simulink library "Math"  (R2023a)
settings: Solver=VariableStepAuto  StartTime=0.0  StopTime=10.0  RelTol=1e-3
libraries: $bdroot x1, simulink x1
settings Model: Creator=FIRSTMentor  LastModifiedBy=FIRSTMentor

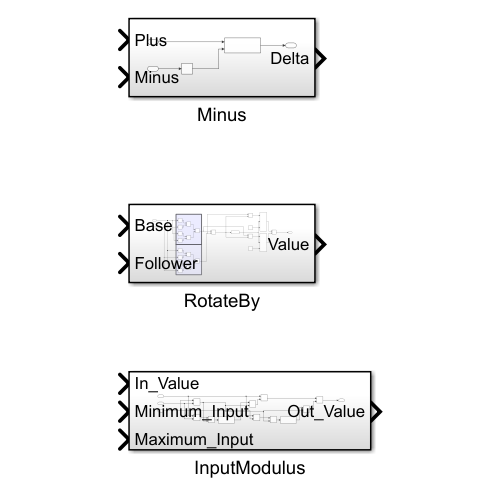
[thumbnail: Simulink's stored preview of the top-level diagram]
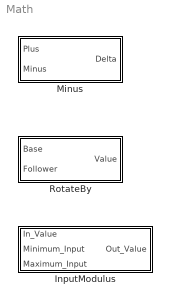
== system Math ==
  InputModulus : Subsystem
  Minus : Subsystem
  RotateBy : Subsystem

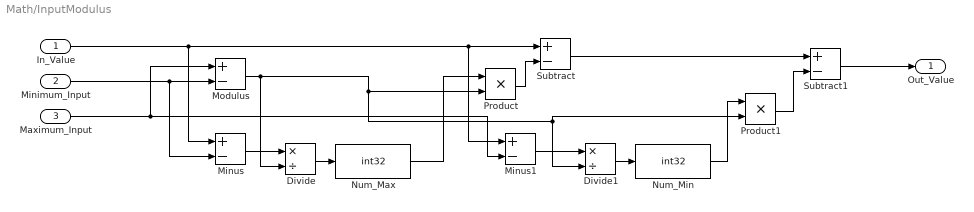
== system Math/InputModulus ==
  In_Value : Inport
  Minimum_Input : Inport  Port=2
  Maximum_Input : Inport  Port=3
  Divide : Product  Inputs=*/
  Divide1 : Product  Inputs=*/
  Minus : Sum  Inputs=+-
  Minus1 : Sum  Inputs=+-
  Modulus : Sum  Inputs=+-
  Num_Max : DataTypeConversion  OutDataTypeStr=int32  SaturateOnIntegerOverflow=off  RndMeth=Floor
  Num_Min : DataTypeConversion  OutDataTypeStr=int32  SaturateOnIntegerOverflow=off  RndMeth=Floor
  Product : Product
  Product1 : Product
  Subtract : Sum  Inputs=+-
  Subtract1 : Sum  Inputs=+-
  Out_Value : Outport
  wires:
  In_Value/1 -> Minus/1, Minus1/1, Subtract/1
  Minimum_Input/1 -> Minus/2, Modulus/2
  Subtract/1 -> Subtract1/1
  Subtract1/1 -> Out_Value/1
  Product/1 -> Subtract/2
  Product1/1 -> Subtract1/2
  Modulus/1 -> Divide/2, Divide1/2, Product1/2, Product/2
  Num_Min/1 -> Product1/1
  Num_Max/1 -> Product/1
  Divide/1 -> Num_Max/1
  Divide1/1 -> Num_Min/1
  Minus1/1 -> Divide1/1
  Minus/1 -> Divide/1
  Maximum_Input/1 -> Minus1/2, Modulus/1

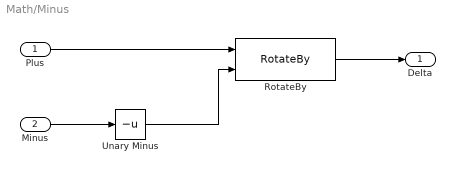
== system Math/Minus ==
  Plus : Inport
  Minus : Inport  Port=2
  RotateBy : $bdroot/RotateBy  SystemSampleTime=-1  VariantActivationTime=update diagram  Latency=0  AutoFrameSizeCalculation=off
  Unary Minus : UnaryMinus
  Delta : Outport
  wires:
  Plus/1 -> RotateBy/1
  RotateBy/1 -> Delta/1
  Minus/1 -> Unary Minus/1
  Unary Minus/1 -> RotateBy/2

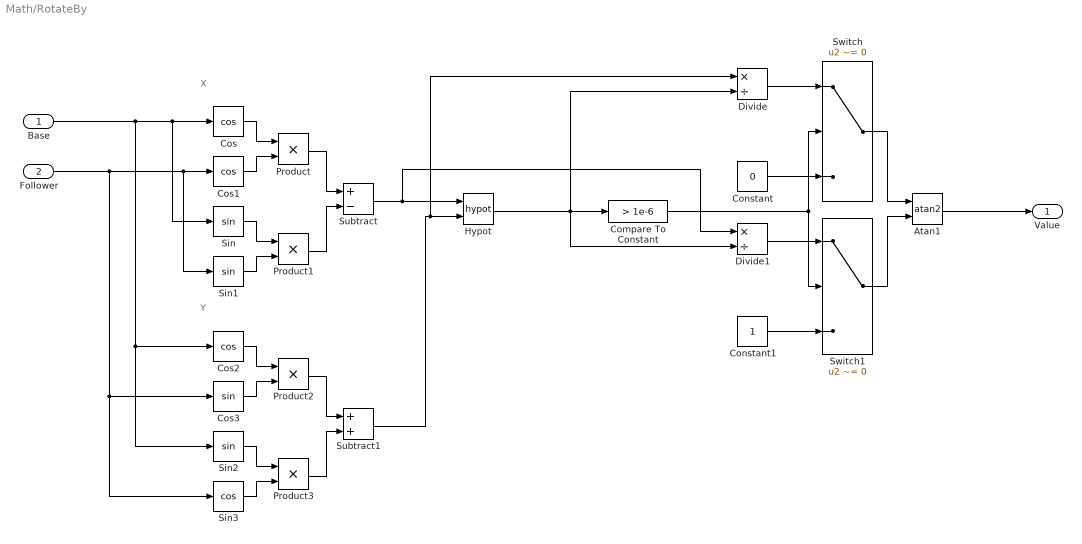
== system Math/RotateBy ==
  note: Y
  note: X
  Base : Inport  OutDataTypeStr=double  Unit=rad
  Follower : Inport  Port=2  OutDataTypeStr=double  Unit=rad
  Atan1 : Trigonometry  Operator=atan2
  Compare To Constant : simulink/Logic and Bit Operations/Compare To Constant  relop=>  const=1e-6  OutDataTypeStr=boolean
  Constant : Constant  Value=0
  Constant1 : Constant
  Cos : Trigonometry  Operator=cos
  Cos1 : Trigonometry  Operator=cos
  Cos2 : Trigonometry  Operator=cos
  Cos3 : Trigonometry
  Divide : Product  Inputs=*/
  Divide1 : Product  Inputs=*/
  Hypot : Math  Operator=hypot
  Product{,1..3} (4 alike) : Product
  Sin : Trigonometry
  Sin1 : Trigonometry
  Sin2 : Trigonometry
  Sin3 : Trigonometry  Operator=cos
  Subtract : Sum  Inputs=+-
  Subtract1 : Sum
  Switch : Switch  Criteria=u2 ~= 0  SaturateOnIntegerOverflow=off  InputSameDT=off
  Switch1 : Switch  Criteria=u2 ~= 0  SaturateOnIntegerOverflow=off  InputSameDT=off
  Value : Outport  OutDataTypeStr=double  Unit=rad
  wires:
  Base/1 -> Sin2/1, Cos2/1, Sin/1, Cos/1
  Follower/1 -> Sin3/1, Cos3/1, Sin1/1, Cos1/1
  Cos/1 -> Product/1
  Cos1/1 -> Product/2
  Sin/1 -> Product1/1
  Sin1/1 -> Product1/2
  Product/1 -> Subtract/1
  Product1/1 -> Subtract/2
  Cos3/1 -> Product2/2
  Sin3/1 -> Product3/2
  Product2/1 -> Subtract1/1
  Cos2/1 -> Product2/1
  Product3/1 -> Subtract1/2
  Sin2/1 -> Product3/1
  Atan1/1 -> Value/1
  Subtract/1 -> Divide1/1, Hypot/1
  Subtract1/1 -> Divide/1, Hypot/2
  Hypot/1 -> Divide1/2, Divide/2, Compare To Constant/1
  Switch/1 -> Atan1/1
  Switch1/1 -> Atan1/2
  Constant/1 -> Switch/3
  Constant1/1 -> Switch1/3
  Compare To Constant/1 -> Switch1/2, Switch/2
  Divide/1 -> Switch/1
  Divide1/1 -> Switch1/1
